simulink model "PrismaticControl"  (R2019b)
settings: Solver=VariableStepAuto  StartTime=0.0  StopTime=10  RelTol=1e-3
undefined symbols (not defined in the file or in its folder): X, Y, Z
libraries: fl_lib x72, nesl_utility x38, sm_lib x28, fl_ps_legacy_lib x16, ee_lib x11, simulink x5, simulink_extras x4
(part 3 of 3)

== system PrismaticControl/STEPPER 2 CONTROL/Controller/Speed/Step Rate and Direction/IC Analog Output Vref ==
  SL : Inport
  Controlled Voltage Source : fl_lib/Electrical/Electrical Sources/Controlled Voltage Source
  ERef : fl_lib/Electrical/Electrical Elements/Electrical Reference
  Simulink-PS Converter : nesl_utility/Simulink-PS Converter  PhysicalDomain=network_engine_domain  SubClassName=ps_input  LeftPortType=input  RightPortType=output  PseudoPeriodic=off  Frequencies=[]  NoiseDistribution=none  NoiseParameters=[]  Unit=V  AffineConversion=off  FilteringAndDerivatives=zero  SimscapeFilterOrder=1  InputFilterTimeConstant=.001  UdotUserProvided=0
  V : PMIOPort  Side=Right
  wires:
  SL/1 -> Simulink-PS Converter/1
  connections:
  ERef/LConn1 -- Controlled Voltage Source/RConn2
  V/RConn1 -- Controlled Voltage Source/LConn1
  Simulink-PS Converter/RConn1 -- Controlled Voltage Source/RConn1

== system PrismaticControl/STEPPER 1 CONTROL/Controller1/Position/Algorithm and Pulse Generation/Pulse Generator/Pulse Generator ==
  -1 : Gain  Gain=0.5
  Constant : Constant  SampleTime=1/(2*f)
  Gain : Gain  Gain=-1
  Sum : Sum  Inputs=|++
  "Unit Delay, sample time 1/2*f)" : UnitDelay  InitialCondition=-1  SampleTime=1/(2*f)  HasFrameUpgradeWarning=on
  p : Outport  VectorParamsAs1DForOutWhenUnconnected=off
  wires:
  "Unit Delay, sample time 1/2*f)"/1 -> Gain/1, Sum/1
  Gain/1 -> "Unit Delay, sample time 1/2*f)"/1
  Constant/1 -> Sum/2
  Sum/1 -> -1/1
  -1/1 -> p/1

== matlab function PrismaticControl/Coordinate conversion1 ==
  data: azimuth input; x output; elevation input; r input; y output; z output
function [x, y, z] = fcn(azimuth,elevation,r)

 azimuth = deg2rad(azimuth);
 elevation = deg2rad(elevation);
[x, y, z] = sph2cart(azimuth,elevation,r);

end

== matlab function PrismaticControl/Coordinate conversion ==
  data: x input; azimuth output; y input; z input; elevation output; r output
function [azimuth,elevation,r] = fcn(x, y, z)

    [azimuth,elevation,r] = cart2sph(x,y,z);
    azimuth = rad2deg(azimuth);
    elevation = rad2deg(elevation);
end
